simulink model "narmaL2"  (R2018b)
settings: Solver=ode45  StartTime=0.0  StopTime=600  RelTol=1e-3  AbsTol=1e-8  EnableMultiTasking=on
undefined symbols (not defined in the file): Ar, hmax, k12, k2, qmax, qmin
libraries: neural x1
settings Model: Creator=Adolfo  LastModifiedBy=Abdullah
settings SolverCC: AutoScaleAbsTol=off
settings DataIOCC: LimitDataPoints=on  SaveFormat=Array  SignalLoggingSaveFormat=ModelDataLogs
settings OptimizationCC: ExpressionDepthLimit=2147483647  InitFltsAndDblsToZero=on  LifeSpan=inf
settings DebuggingCC: SaveWithParameterizedLinksMsg=none  UnderspecifiedInitializationDetection=Classic  MergeDetectMultiDrivingBlocksExec=none  SignalResolutionControl=TryResolveAllWithWarning  SolverPrmCheckMsg=warning  MultiTaskDSMMsg=warning  MultiTaskCondExecSysMsg=none  FcnCallInpInsideContextMsg=warning  StateNameClashWarn=warning  SFUnexpectedBacktrackingDiag=warning  SFNoUnconditionalDefaultTransitionDiag=warning  SFExecutionAtInitializationDiag=none
settings HardwareCC: ProdBitPerPointer=32  ProdBitPerSizeT=32  ProdBitPerPtrDiffT=32  ProdLargestAtomicFloat=None  ProdIntDivRoundTo=Undefined  ProdEndianess=Unspecified  ProdWordSize=32  ProdHWDeviceType=32-bit Generic
settings ModelReferenceCC: PropagateSignalLabelsOutOfModel=off
settings SFSimCC: SimUseLocalCustomCode=off
settings RTWCC: RTWUseLocalCustomCode=off
settings CodeAppCC: StateflowObjectComments=on
settings GRTTargetCC: TargetFcnLib=ansi_tfl_tmw.mat  TargetLangStandard=C89/C90 (ANSI)  GeneratePreprocessorConditionals=Disable all  CombineOutputUpdateFcns=off  GRTInterface=on
settings ConfigComp: CovMetricSettings=dw  CovHtmlReporting=on  CovSaveCumulativeToWorkspaceVar=on  CovSaveSingleToWorkspaceVar=on  CovExternalEMLEnable=off

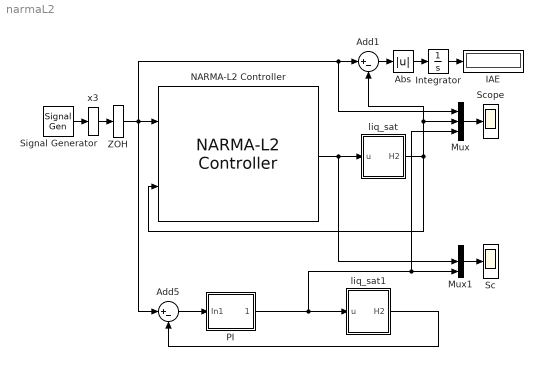
== system narmaL2 ==
  Abs : Abs
  Add1 : Sum  Inputs=|+-
  Add5 : Sum  Inputs=|+-
  IAE : Display
  Integrator : Integrator
  Mux : Mux  Inputs=3
  Mux1 : Mux  Inputs=3
  NARMA-L2 Controller : neural/Control Systems/NARMA-L2 Controller  Normalize=1  IW1_1=[0.53747767708707250289 0.18099511930578765506 -0.34314137000612848771 0.23876517762648577503 0.50383873296237657868 -0.43639354717711442699 -0.055956388088357289501 0.30206751105676726832 0.037521207664510301816 0.16207018017815774669 0.55827365279958363065;0.19300591445248951872 0.25485699956780083486 0.23863059122897428699 0.167814079529104071 0.39275238511665910845 0.30674901632643863936 0.04964530812044430641 -0.038947246947648936355 0.30620507408718439235 0.72642765396046682369 0.49710007769989611459;-0.0948507230021711778 -0.10173116498504017335 0.0021321759584975608776 0.11341173147666640253 0.019191540040389188509 0.12950564378493334416 -0.056952604569590420391 0.030487222422210125822 0.0004446037806052112332 0.11863774823057748886 0.15595009018127908851;1.0568439816849815038 -1.1891615073426782256 -0.75162148248571902798 0.052772407578153546215 0.047324810445031319228 -0.26029855799446549591 0.49543899549102315971 -0.3380945780364931208 -0.23364921917912548355 -0.29811688046211398673 -0.67511710476270614389;0.26055730223984446825 0.28154251692045612065 0.090013242258030617959 -0.057711260918890547322 0.0099225655439794703538 -0.0032943630554241923845 -0.19141834829601400703 -0.26363144057994319924 -0.25407858196768567938 -0.043627192667109716828 0.051239160988922539952;-0.013014437274007273695 0.29860475973668493266 0.027229819683618733395 -0.020950185250509942292 0.075951934788676817023 0.2130185947607864394 0.024789294314940351488 0.20138353790252144782 -0.009189834023158309495 0.67865817966829800056 0.20959487422525077682;0.4103555182995822781 0.045385991503774571199 0.19057180129406611768 0.094208565624253018389 -0.025425947305399293485 -0.18867466322845807825 -0.10772412718192429792 0.15817410030447706659 0.15760449312450608428 -0.035303661996994493977 -0.17168064124945525695;-0.073961887385569510811 0.0654154716181726964 -0.084333422138595140471 -0.075385313564872005743 -0.10794785629639097602 0.0059518773506479893259 -0.068432043619970378545 0.06068728297616821088 0.22008611559842899963 0.2172072078351281188 0.054130639281553975806;0.020125373455329671757 -0.11961574014843032177 0.2240341060373241544 -0.010032879332567842812 0.22399039823982899722 0.45094290718451501832 -0.13727773995166467347 -0.17931084057615653826 0.33501847057556682907 -0.35179542068878510985 0.13238320672551193158;-0.28300713551783734934 -0.018507914062523452003 0.13945581204644769135 0.40688513837425033248 -0.059786204521418834235 -0.41353202284523976617 -0.095252783498966667186 0.20141901185373015104 0.45544080235018957747 -0.20596876962194027305 -0.25723801943258378655;0.054179507072483860941 0.093958563154519822436 0.1440805976146098677 0.084655009732686747892 0.026792651581584493031 0.17809838471981234709 0.054007705997900876116 0.17565512184113932226 0.59006575011241813034 0.87391955133141285827 0.86392832578145595246;0.29915455134824742167 0.066999922117568291857 -0.023170591200176844648 0.16527073192479732611 0.058796448288032952811 -0.22009330594340870135 0.21411839523847606137 0.5586801900396214382 0.39541856812544795563 -0.3400213507484781128 -0.051667621960224452415;-0.9623589751325695163 0.6327576917604661455 -0.1246078138397020002 -0.010177860140266309363 0.0091378587858966051766 0.087151622712129062087 -0.01847307441225331387 -0.041510581968375245832 0.031677587763874109905 -0.018089429932786615929 0.016555530037445510827;1.1848325426350876377 1.0068492805920106203 0.95664785672172347741 0.49086293245865103563 0.19599133611179886394 0.046018614366887589107 0.12394112321407027566 0.031991681352900556978 0.50369623416211772859 0.26537777995476541371 0.54661292435929931255;0.29965514207875448838 0.47173870702917874986 0.60655788497052798292 0.64595866798671675024 0.73247474848576421547 0.64252763195289397391 0.56481767009427519266 0.78086465137275340442 -0.55822976296440218746 0.0026644311568674722279 0.021387352899476439611]  IW3_2=[-0.035593782198517290305 -0.22160467087487231708 -0.33780560153558714109 -0.2873111401829575029 -0.21503221939142566632 -0.23990888802504597987 0.13832874002683787085 0.03854927844967216688 -0.99002920583462983295 0.25307359094881476391 -0.25390896766296761067;0.28780535976996035608 0.15504126195904852081 0.35022428665310606499 0.20413700381130880923 0.14172766141069112478 0.037042874318195542771 0.0904595706421410517 -0.066703367166699542579 0.77754159477550510715 0.096849824311934881726 0.26641902758620789049;-0.18395580199587527326 -0.096432338620644195148 0.010761228434170478502 -0.13391375737973379434 0.026950204740516490315 0.013683629538897120609 0.16361002789496773002 0.50964477378531536367 -0.55180358840805354692 0.098864261529533106754 -0.48466381038846717555;-0.091508931330164910989 0.17793144801983040715 0.35472960483490878492 0.68495740422883888421 0.64098872302511689103 0.39440192401978801939 0.36034736483106921678 -0.25957782720442706959 -0.08369936454337464915 -0.34801488399904845217 -0.39580857087238885406;1.1887938706535627897 0.52745766996003506932 0.13098109610337005382 0.13348139807770184606 -0.034512037249875629485 -0.26048441990403814472 -0.12718314394622723396 0.16582496350912534488 0.25389403376264646495 -0.23029759366848648328 -0.29594621696800538224;0.74297824902908293776 0.59956916530282022837 0.67658685488962411192 0.59339957376154139901 0.52933056401510014677 -0.17488151510027089008 0.021461099539255228119 -0.38068417839967222394 1.5386382880332707401 0.027759912720403241704 -0.16343636571017877701;0.039668532021102549667 0.039660974521482844635 0.021645116559085592761 0.057853060257847456482 -0.26582547307462056629 -0.51759219833417124956 -0.51821334892033066311 -0.40244167971211924906 -1.2861162738679874362 0.49556978851963578991 -0.059610383168827635325;-0.069877947774947421489 -0.2271137264629810304 -0.040763891063289064975 0.10969991388600607018 -0.04336860480553157704 0.19160044543971638253 0.66713760117605602762 0.19534096190897698442 0.04455715121352880892 0.57355653527457195473 1.7050777654994768717;0.34554457143088107562 0.26174557244344404117 0.33243081316843881012 0.17898062486547444694 0.083211875630810672178 -0.20159722084743256221 -0.15014874951230411382 -0.045782257001895011739 0.048673087556522380559 0.21175955589561634707 -0.093389565797441731476;0.31842402771214606272 0.2451229649688464185 0.017880669834881450508 -0.051259372978931121156 -0.33269117585318153107 -0.18992568937561626896 0.076862062620842677707 -0.44364753918580229763 -0.31221335851317449928 -0.28428757132902915394 0.11725969694138291266;-0.62785408390734132045 -0.33937714156820375511 -0.53101420228490081588 -0.65393327631778452869 -0.63316383660636854636 -0.51006428522351121568 -0.23980247178153002441 -0.1304403703590295005 1.473969748133704627 -0.44562177575402689422 -0.64992167540147449678;-0.11925001912794634673 -0.096178754860089463175 0.071757770848605934022 0.01785245846120548166 0.13673455601567921502 0.039402466643050262918 0.19382823760806158764 0.096173529874912316862 0.058383344380386600903 0.20249032442551248567 0.27182541579381719332;0.16545317473243320583 0.28439275640642824872 0.10045326853734401484 0.24101546050332281479 0.010410109001065620538 -0.069474822053575413516 0.063483290289172558674 -0.12199924479364153418 -0.32427518451536668787 -0.20179165421692857318 0.42236909890798834954;-0.065058005771503585324 0.094028224063650800435 0.045526138707431107466 0.11714456596247076192 0.22268844813947824557 0.33077295457820932167 0.43491144749751892151 0.36838323006075701649 -0.02264512227795507926 -0.25191215178301340494 0.052767190154927118284;0.50843110162768334614 0.4201511020863483159 0.54961773522985313267 0.41776210579813144452 0.33227214841598412542 0.099819991958263215581 0.35429717620654238575 -0.0041481970703330754702 -0.81441364890623135775 0.67348277553381974414 -0.63215597454934069344]  IW5_3=0.34445710162019838041  LW2_1=[-1.4546182360464723349 0.3114393249868889213 0.36551891478241127498 -1.5006268461931155933 -0.21155968139285977192 -0.43991068763880808445 1.9021191345026167152 -0.43414421301555372601 0.90960840718896485146 -1.4162709575119090122 0.006989096350229371743 -0.12250656041425427023 -8.8157453870185147338 -0.022200102606832184532 -0.015609102123666814335]  LW4_3=[2.1092235734619091403 0.83475569673400507043 0.84186976839022353847 -0.82700643882994018252 1.3314393402187907345 2.0420330644900581696 1.0689422192939666001 1.4075940580409433966 -0.32066487542105026609 0.74543752556504305762 -0.10229922218763785879 0.10560638006712570747 2.5310271655940126401 0.21693546446512645964 1.1119468840039392621]  LW5_4=-0.30062700464664787736  LW6_5=0.27691269933043033413  LW6_2=0.22150615616318680701  B1=[-1.7569172750104702363;-0.98437931162619296543;2.6470267398758724475;2.1823783651091011038;-2.0312774712712826641;-0.33546031458547115323;0.86404555964318419115;3.550950223447927101;-0.06751594682054785912;-0.53912901064871088241;1.2368930417100889585;1.656921413139981869;0.19955993636368829502;-1.0276491673694081452;0.22751930298456699009]  B2=-0.02774242571397469298  B3=[-2.1979538614458209445;1.9834584613223693594;-4.5033878951745700547;-1.5052903376245945211;1.4201605156583498868;-2.8893478051215506497;1.4123830551560963009;-2.5750849211930253446;4.4214970527878838524;-0.35750752661236301355;-1.0097550949020885902;2.3418997275193715879;-2.6875090761214921464;2.3295561158220658982;-1.5481680398189321402]  B4=1.8488586159660946873  Limit_output=0  min_output=-Inf  max_output=Inf  Use_Previous_Weights=1  Ts=10  S1=15  Ni=4  Nj=8  sim_file=mod_liq2  trainfun=trainlm  Use_validation=1  Use_Testing=1  max_i=90  min_i=0  max_i_int=400  min_i_int=1  sam_training=1500  epochs=500  minp=0.11887020659804403699  maxp=89.256193015686704939  mint=0  maxt=89.256193015686704939
      settings: SourceProductName=Deep Learning Toolbox  SourceProductBaseCode=NN
  PI : Subsystem
  Sc : Scope
  Scope : Scope
  Signal Generator : SignalGenerator  WaveForm=square  Amplitude=-12/300  Frequency=1/600
  ZOH : ZeroOrderHold  SampleTime=100
  liq_sat : Subsystem
  liq_sat1 : Subsystem
  x3 : Integrator
  wires:
  Mux/1 -> Scope/1
  NARMA-L2 Controller/1 -> Mux1/2, liq_sat/1(u)
  PI/1(Out1) -> Mux/3, Mux1/3, liq_sat1/1(u)
  Add5/1 -> PI/1(In1)
  Mux1/1 -> Sc/1
  liq_sat1/1(H2) -> Add5/2
  liq_sat/1(H2) -> Mux/2, Add1/2, NARMA-L2 Controller/2
  Signal Generator/1 -> x3/1
  x3/1 -> ZOH/1
  ZOH/1 -> Add5/1, Mux/1, Add1/1, NARMA-L2 Controller/1
  Add1/1 -> Abs/1
  Abs/1 -> Integrator/1
  Integrator/1 -> IAE/1

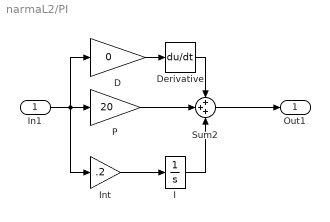
== system narmaL2/PI ==
  In1 : Inport
  D : Gain  Gain=0
  Derivative : Derivative
  I : Integrator
  Int : Gain  Gain=.2
  P : Gain  Gain=20
  Sum2 : Sum  Inputs=+++
  Out1 : Outport
  wires:
  In1/1 -> P/1, Int/1, D/1
  P/1 -> Sum2/2
  I/1 -> Sum2/3
  Sum2/1 -> Out1/1
  Int/1 -> I/1
  D/1 -> Derivative/1
  Derivative/1 -> Sum2/1

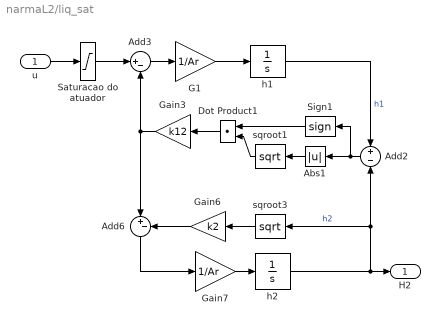
== system narmaL2/liq_sat ==
  u : Inport
  Abs1 : Abs
  Add2 : Sum  Inputs=+-
  Add3 : Sum  Inputs=|+-
  Add6 : Sum  Inputs=|+-
  Dot Product1 : DotProduct  InputSameDT=on  OutDataTypeStr=Inherit: Inherit via internal rule
  G1 : Gain  Gain=1/Ar
  Gain3 : Gain  Gain=k12
  Gain6 : Gain  Gain=k2
  Gain7 : Gain  Gain=1/Ar
  Saturacao do atuador : Saturate  UpperLimit=qmax  LowerLimit=qmin
  Sign1 : Signum
  h1 : Integrator  LimitOutput=on  UpperSaturationLimit=hmax  LowerSaturationLimit=0
  h2 : Integrator  LimitOutput=on  UpperSaturationLimit=hmax  LowerSaturationLimit=0
  sqroot1 : Math  Operator=sqrt  SaturateOnIntegerOverflow=on
  sqroot3 : Math  Operator=sqrt  SaturateOnIntegerOverflow=on
  H2 : Outport
  wires:
  h1/1 -> Add2/1  "h1"
  h2/1 -> Add2/2, sqroot3/1, H2/1  "h2"
  Saturacao do atuador/1 -> Add3/1
  Add6/1 -> Gain7/1
  Gain6/1 -> Add6/2
  Gain7/1 -> h2/1
  sqroot3/1 -> Gain6/1
  G1/1 -> h1/1
  Gain3/1 -> Add6/1, Add3/2
  Add3/1 -> G1/1
  Dot Product1/1 -> Gain3/1
  sqroot1/1 -> Dot Product1/2
  Sign1/1 -> Dot Product1/1
  Abs1/1 -> sqroot1/1
  Add2/1 -> Abs1/1, Sign1/1
  u/1 -> Saturacao do atuador/1

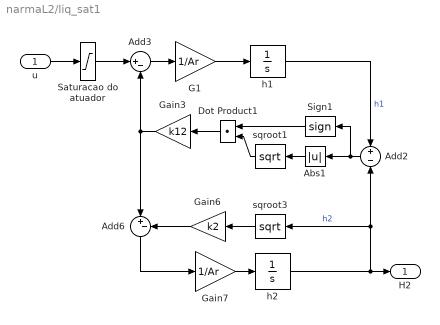
== system narmaL2/liq_sat1 ==
  u : Inport
  Abs1 : Abs
  Add2 : Sum  Inputs=+-
  Add3 : Sum  Inputs=|+-
  Add6 : Sum  Inputs=|+-
  Dot Product1 : DotProduct  InputSameDT=on  OutDataTypeStr=Inherit: Inherit via internal rule
  G1 : Gain  Gain=1/Ar
  Gain3 : Gain  Gain=k12
  Gain6 : Gain  Gain=k2
  Gain7 : Gain  Gain=1/Ar
  Saturacao do atuador : Saturate  UpperLimit=qmax  LowerLimit=qmin
  Sign1 : Signum
  h1 : Integrator  LimitOutput=on  UpperSaturationLimit=hmax  LowerSaturationLimit=0
  h2 : Integrator  LimitOutput=on  UpperSaturationLimit=hmax  LowerSaturationLimit=0
  sqroot1 : Math  Operator=sqrt  SaturateOnIntegerOverflow=on
  sqroot3 : Math  Operator=sqrt  SaturateOnIntegerOverflow=on
  H2 : Outport
  wires:
  h1/1 -> Add2/1  "h1"
  h2/1 -> Add2/2, sqroot3/1, H2/1  "h2"
  Saturacao do atuador/1 -> Add3/1
  Add6/1 -> Gain7/1
  Gain6/1 -> Add6/2
  Gain7/1 -> h2/1
  sqroot3/1 -> Gain6/1
  G1/1 -> h1/1
  Gain3/1 -> Add6/1, Add3/2
  Add3/1 -> G1/1
  Dot Product1/1 -> Gain3/1
  sqroot1/1 -> Dot Product1/2
  Sign1/1 -> Dot Product1/1
  Abs1/1 -> sqroot1/1
  Add2/1 -> Abs1/1, Sign1/1
  u/1 -> Saturacao do atuador/1
